simulink model "KinematicControl_CBF_cvxpy"  (R2024a)
settings: Solver=FixedStepAuto  StartTime=0.0  StopTime=Tf  FixedStep=Ts  RelTol=1e-3
undefined symbols (not defined in the file): config, d, gamma, InitAng, InitPos, lambda, Ts, x_obs
libraries: robotmaniplib x3, matrix_library x2, slctrl_constraint x1
settings Model: Creator=bumyong  LastModifiedBy=bumyong

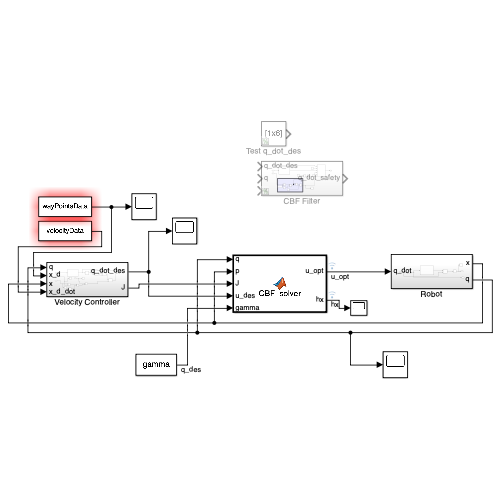
[thumbnail: Simulink's stored preview of the top-level diagram]
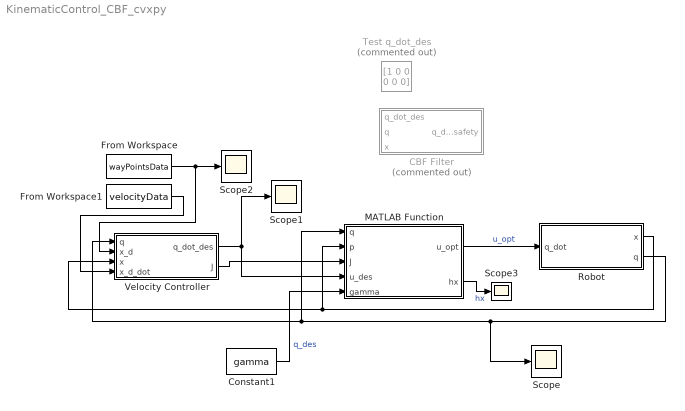
== system KinematicControl_CBF_cvxpy ==
  CBF Filter : Subsystem  Commented=on
  Constant1 : Constant  Value=gamma
  From Workspace : FromWorkspace  VariableName=wayPointsData  Interpolate=off  OutputAfterFinalValue=Holding final value
  From Workspace1 : FromWorkspace  VariableName=velocityData  Interpolate=off  OutputAfterFinalValue=Holding final value
  MATLAB Function : MATLAB Function  TreatAsAtomicUnit=on
  Robot : Subsystem
  Scope{,1..3} (4 alike) : Scope
  Test q_dot_des : Constant  Commented=on  Value=[1 0 0 0 0 0]
  Velocity Controller : Subsystem
  wires:
  Velocity Controller/1(q_dot_des) -> MATLAB Function/4(u_des), Scope1/1
  Robot/1(x) -> MATLAB Function/2(p), Velocity Controller/3(x)
  From Workspace/1 -> Velocity Controller/2(x_d), Scope2/1
  From Workspace1/1 -> Velocity Controller/4(x_d_dot)
  Robot/2(q) -> Scope/1, MATLAB Function/1(q), Velocity Controller/1(q)
  Constant1/1 -> MATLAB Function/5(gamma)  "q_des"
  Velocity Controller/2(J) -> MATLAB Function/3(J)
  MATLAB Function/1(u_opt) -> Robot/1(q_dot)  "u_opt"
  MATLAB Function/2(hx) -> Scope3/1  "hx"

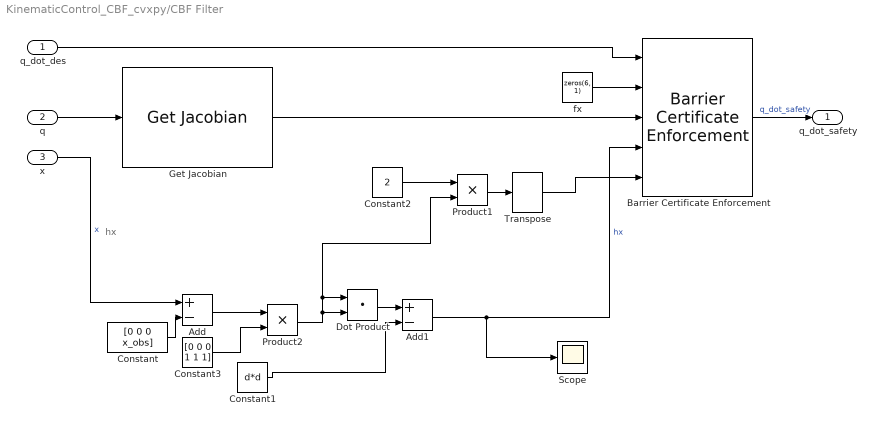
== system KinematicControl_CBF_cvxpy/CBF Filter ==
  note: hx
  q_dot_des : Inport
  q : Inport  Port=2
  x : Inport  Port=3
  Add : Sum  Inputs=+-
  Add1 : Sum  Inputs=+-
  Barrier Certificate Enforcement : slctrl_constraint/Barrier Certificate Enforcement  nx=6  nu=6  nc=1  gamma=gamma  beta=1  external_umax=off  external_umin=off  Ts=Ts  maxiter=200  tol=1e-6  output_exitflag=off
      settings: LibrarySourceBlock=slctrlblks/Constraint Control/Barrier Certificate Enforcement
  Constant : Constant  Value=[0 0 0 x_obs]
  Constant1 : Constant  Value=d*d
  Constant2 : Constant  Value=2
  Constant3 : Constant  Value=[0 0 0 1 1 1]
  Dot Product : DotProduct  OutDataTypeStr=Inherit: Inherit via internal rule
  Get Jacobian : robotmaniplib/Get Jacobian  RigidBodyTree=robot  EndEffector=link7  SimulateUsing=Interpreted execution
  Product1 : Product
  Product2 : Product
  Scope : Scope
  Transpose : matrix_library/Transpose
  fx : Constant  Value=zeros(6, 1)
  q_dot_safety : Outport
  wires:
  q_dot_des/1 -> Barrier Certificate Enforcement/1
  fx/1 -> Barrier Certificate Enforcement/2
  Barrier Certificate Enforcement/1 -> q_dot_safety/1  "q_dot_safety"
  Add1/1 -> Scope/1, Barrier Certificate Enforcement/4  "hx"
  Dot Product/1 -> Add1/1
  Constant1/1 -> Add1/2
  Get Jacobian/1 -> Barrier Certificate Enforcement/3
  Constant/1 -> Add/2
  q/1 -> Get Jacobian/1
  Constant2/1 -> Product1/1
  Product1/1 -> Transpose/1
  Transpose/1 -> Barrier Certificate Enforcement/5
  x/1 -> Add/1  "x"
  Add/1 -> Product2/1
  Product2/1 -> Dot Product/2, Product1/2, Dot Product/1
  Constant3/1 -> Product2/2

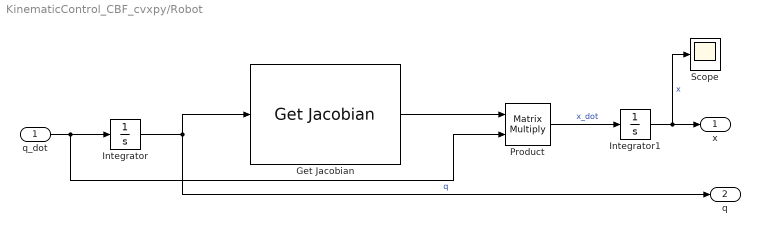
== system KinematicControl_CBF_cvxpy/Robot ==
  q_dot : Inport
  Get Jacobian : robotmaniplib/Get Jacobian  RigidBodyTree=robot  EndEffector=link7  SimulateUsing=Interpreted execution
  Integrator : Integrator  InitialCondition=config
  Integrator1 : Integrator  InitialCondition=[InitAng, InitPos]'
  Product : Product  Multiplication=Matrix(*)
  Scope : Scope
  x : Outport
  q : Outport  Port=2
  wires:
  q_dot/1 -> Product/2, Integrator/1
  Integrator/1 -> q/1, Get Jacobian/1  "q"
  Get Jacobian/1 -> Product/1
  Product/1 -> Integrator1/1  "x_dot"
  Integrator1/1 -> Scope/1, x/1  "x"

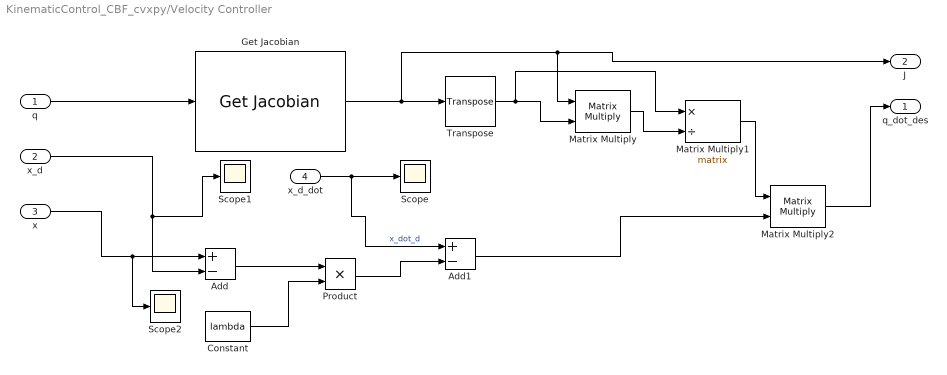
== system KinematicControl_CBF_cvxpy/Velocity Controller ==
  q : Inport
  x_d : Inport  Port=2
  x : Inport  Port=3
  x_d_dot : Inport  Port=4
  Add : Sum  Inputs=+-
  Add1 : Sum  Inputs=+-
  Constant : Constant  Value=lambda
  Get Jacobian : robotmaniplib/Get Jacobian  RigidBodyTree=robot  EndEffector=link7  SimulateUsing=Interpreted execution
  Matrix Multiply : Product  Multiplication=Matrix(*)
  Matrix Multiply1 : Product  Inputs=*/  Multiplication=Matrix(*)
  Matrix Multiply2 : Product  Multiplication=Matrix(*)
  Product : Product
  Scope : Scope
  Scope1 : Scope
  Scope2 : Scope
  Transpose : matrix_library/Transpose
  q_dot_des : Outport
  J : Outport  Port=2
  wires:
  q/1 -> Get Jacobian/1
  Get Jacobian/1 -> J/1, Matrix Multiply/1, Transpose/1
  Transpose/1 -> Matrix Multiply1/1, Matrix Multiply/2
  Matrix Multiply/1 -> Matrix Multiply1/2
  x_d/1 -> Scope1/1, Add/2
  x/1 -> Scope2/1, Add/1
  Add/1 -> Product/1
  Constant/1 -> Product/2
  x_d_dot/1 -> Add1/1, Scope/1  "x_dot_d"
  Product/1 -> Add1/2
  Add1/1 -> Matrix Multiply2/2
  Matrix Multiply1/1 -> Matrix Multiply2/1
  Matrix Multiply2/1 -> q_dot_des/1

== matlab function KinematicControl_CBF_cvxpy/MATLAB Function ==
  data: q input; u_opt output; p input; J input; u_des input; gamma input; hx output
function [u_opt, hx]  = CBF_solver(q, p, J, u_des, gamma)

    u_opt = double([0 0 0 0 0 0]');
    hx = double(0);

    p_obs = [0 0.45 0.2]'; % Position of the obstacle
    R = 0.15; % Radious of the obstacle
    R_w = 0.05; % Radious of the wrist of robot

    coder.extrinsic('py.KinematicControl_CBF_cvxpy.manipulator_cbf');


    result = py.KinematicControl_CBF_cvxpy.manipulator_cbf(q, p(4:6), J, u_des, gamma);
    hx = norm(p(4:6) - p_obs)^2 - (R + R_w)^2;

    u_opt = double(result)';
end
